simulink model "kalman_estimate_MM"  (R2018b)
settings: Solver=FixedStepAuto  StartTime=0.0  StopTime=500  FixedStep=0.02  RelTol=1e-3
values from neighbouring files (symbols this model uses):
  D = randn(num_output,num_control)    [Com_of_linear_model_calculate.m]    (also in Copy_of_linear_model_calculate.m; D.mat = [0 0 0.00507528406191 0.0236369284061 0.221173094143 0.00198; LINEAR.m = randn(8,1)*10; MM_HKF.m = reshape(out(A_l+B_l+C_l+1:A_l+B_l+C_l+D_l),size_D))
undefined symbols (not defined in the file or in its folder): act_piece, com_piece, piece, sigbuilder_block
libraries: sharedschedule x467, dspsigattribs x44, commchan3 x1
(part 4 of 5)

== system kalman_estimate_MM/sen3_PWL-model ==
  u : Inport
  x0 : Inport  Port=2
  A : sharedschedule/Interpolate Matrix(x)   matrix=sen3_piece.A  aMode=aMode
      settings: SourceProductName=Aerospace Blockset  SourceProductBaseCode=AE
  Add : Sum
  B : sharedschedule/Interpolate Matrix(x)   matrix=sen3_piece.B  aMode=aMode
      settings: SourceProductName=Aerospace Blockset  SourceProductBaseCode=AE
  C : sharedschedule/Interpolate Matrix(x)   matrix=sen3_piece.C  aMode=aMode
      settings: SourceProductName=Aerospace Blockset  SourceProductBaseCode=AE
  D : sharedschedule/Interpolate Matrix(x)   matrix=sen3_piece.D  aMode=aMode
      settings: SourceProductName=Aerospace Blockset  SourceProductBaseCode=AE
  K : sharedschedule/Interpolate Matrix(x)   matrix=sen3_piece.K  aMode=aMode
      settings: SourceProductName=Aerospace Blockset  SourceProductBaseCode=AE
  Minus1 : Sum  Inputs=+-
  Prelookup : PreLookup  BreakpointsData=sen3_piece.Nl  BreakpointObject=Nl  ExtrapMethod=Linear  UseLastBreakpoint=on  DiagnosticForOutOfRangeInput=Warning
  S : sharedschedule/Interpolate Matrix(x)   matrix=sen3_piece.S  aMode=aMode
      settings: SourceProductName=Aerospace Blockset  SourceProductBaseCode=AE
  Selector : Selector  InputPortWidth=2  IndexOptions=Index vector (dialog)  Indices=[1]  OutputSizes=1
  kalman filter1 : Subsystem
  steadyOutput : sharedschedule/Interpolate Matrix(x)   matrix=sen3_piece.steadyOutput  aMode=aMode
      settings: SourceProductName=Aerospace Blockset  SourceProductBaseCode=AE
  steadyState : sharedschedule/Interpolate Matrix(x)   matrix=sen3_piece.steadyState  aMode=aMode
      settings: SourceProductName=Aerospace Blockset  SourceProductBaseCode=AE
  steadyinput : sharedschedule/Interpolate Matrix(x)   matrix=sen3_piece.steadyInput  aMode=aMode
      settings: SourceProductName=Aerospace Blockset  SourceProductBaseCode=AE
  Out1 : Outport
  Out2 : Outport  Port=2
  wires:
  Add/1 -> Out2/1
  steadyOutput/1 -> Add/2
  u/1 -> Minus1/1
  x0/1 -> kalman filter1/5(x0)
  A/1 -> kalman filter1/1(A)
  steadyinput/1 -> Minus1/2
  kalman filter1/1(X_es) -> Selector/1
  Minus1/1 -> kalman filter1/6(U)
  kalman filter1/2(Y_es) -> Out1/1, Add/1
  C/1 -> kalman filter1/3(C)
  steadyState/1 -> kalman filter1/7(Xtrim)
  Selector/1 -> Prelookup/1
  Prelookup/2 -> B/2, C/2, D/2, steadyOutput/2, steadyinput/2, K/2, S/2, steadyState/2, A/2
  B/1 -> kalman filter1/2(B)
  Prelookup/1 -> A/1, B/1, C/1, D/1, steadyOutput/1, steadyinput/1, steadyState/1, K/1, S/1
  D/1 -> kalman filter1/4(D)

== system kalman_estimate_MM/sen8_PIECE kalman ==
  u : Inport
  y : Inport  Port=2
  x0 : Inport  Port=3
  A : sharedschedule/Interpolate Matrix(x)   matrix=sen8_piece.A  aMode=aMode
      settings: SourceProductName=Aerospace Blockset  SourceProductBaseCode=AE
  B : sharedschedule/Interpolate Matrix(x)   matrix=sen8_piece.B  aMode=aMode
      settings: SourceProductName=Aerospace Blockset  SourceProductBaseCode=AE
  C : sharedschedule/Interpolate Matrix(x)   matrix=sen8_piece.C  aMode=aMode
      settings: SourceProductName=Aerospace Blockset  SourceProductBaseCode=AE
  D : sharedschedule/Interpolate Matrix(x)   matrix=sen8_piece.D  aMode=aMode
      settings: SourceProductName=Aerospace Blockset  SourceProductBaseCode=AE
  K_s : sharedschedule/Interpolate Matrix(x)   matrix=sen8_piece.K  aMode=aMode
      settings: SourceProductName=Aerospace Blockset  SourceProductBaseCode=AE
  MATLAB Function : MATLAB Function  TreatAsAtomicUnit=on
  Minus1 : Sum  Inputs=+-
  Minus5 : Sum  Inputs=+-
  Prelookup : PreLookup  BreakpointsData=sen8_piece.Nl  BreakpointObject=Nl  ExtrapMethod=Linear  UseLastBreakpoint=on  DiagnosticForOutOfRangeInput=Warning
  S : sharedschedule/Interpolate Matrix(x)   matrix=sen8_piece.S  aMode=aMode
      settings: SourceProductName=Aerospace Blockset  SourceProductBaseCode=AE
  Selector : Selector  InputPortWidth=2  IndexOptions=Index vector (dialog)  Indices=[1]  OutputSizes=1
  kalman filter1 : Subsystem
  steadyOutput : sharedschedule/Interpolate Matrix(x)   matrix=sen8_piece.steadyOutput  aMode=aMode
      settings: SourceProductName=Aerospace Blockset  SourceProductBaseCode=AE
  steadyState : sharedschedule/Interpolate Matrix(x)   matrix=sen8_piece.steadyState  aMode=aMode
      settings: SourceProductName=Aerospace Blockset  SourceProductBaseCode=AE
  steadyinput : sharedschedule/Interpolate Matrix(x)   matrix=sen8_piece.steadyInput  aMode=aMode
      settings: SourceProductName=Aerospace Blockset  SourceProductBaseCode=AE
  Out1 : Outport
  Out2 : Outport  Port=2
  Out3 : Outport  Port=3
  wires:
  kalman filter1/3(Y_error) -> MATLAB Function/1(err), Out2/1
  u/1 -> Minus1/1
  y/1 -> Minus5/1
  x0/1 -> kalman filter1/6(x0)
  A/1 -> kalman filter1/1(A)
  steadyOutput/1 -> Minus5/2
  K_s/1 -> kalman filter1/5(K)
  steadyinput/1 -> Minus1/2
  kalman filter1/1(X_es) -> Selector/1
  Minus1/1 -> kalman filter1/8(U)
  kalman filter1/2(Y_es) -> Out1/1
  Minus5/1 -> kalman filter1/7(Y)
  C/1 -> kalman filter1/3(C)
  steadyState/1 -> kalman filter1/9(Xtrim)
  Selector/1 -> Prelookup/1
  Prelookup/2 -> B/2, C/2, D/2, steadyOutput/2, steadyinput/2, K_s/2, S/2, steadyState/2, A/2
  B/1 -> kalman filter1/2(B)
  Prelookup/1 -> A/1, B/1, C/1, D/1, steadyOutput/1, steadyinput/1, steadyState/1, K_s/1, S/1
  D/1 -> kalman filter1/4(D)
  S/1 -> MATLAB Function/2(S)
  MATLAB Function/1(y) -> Out3/1

== system kalman_estimate_MM/sen8_PWL ==
  u : Inport
  x0 : Inport  Port=2
  A : sharedschedule/Interpolate Matrix(x)   matrix=sen8_piece.A  aMode=aMode
      settings: SourceProductName=Aerospace Blockset  SourceProductBaseCode=AE
  Add : Sum
  B : sharedschedule/Interpolate Matrix(x)   matrix=sen8_piece.B  aMode=aMode
      settings: SourceProductName=Aerospace Blockset  SourceProductBaseCode=AE
  C : sharedschedule/Interpolate Matrix(x)   matrix=sen8_piece.C  aMode=aMode
      settings: SourceProductName=Aerospace Blockset  SourceProductBaseCode=AE
  D : sharedschedule/Interpolate Matrix(x)   matrix=sen8_piece.D  aMode=aMode
      settings: SourceProductName=Aerospace Blockset  SourceProductBaseCode=AE
  K : sharedschedule/Interpolate Matrix(x)   matrix=sen8_piece.K  aMode=aMode
      settings: SourceProductName=Aerospace Blockset  SourceProductBaseCode=AE
  Minus1 : Sum  Inputs=+-
  Prelookup : PreLookup  BreakpointsData=sen8_piece.Nl  BreakpointObject=Nl  ExtrapMethod=Linear  UseLastBreakpoint=on  DiagnosticForOutOfRangeInput=Warning
  S : sharedschedule/Interpolate Matrix(x)   matrix=sen8_piece.S  aMode=aMode
      settings: SourceProductName=Aerospace Blockset  SourceProductBaseCode=AE
  Selector : Selector  InputPortWidth=2  IndexOptions=Index vector (dialog)  Indices=[1]  OutputSizes=1
  kalman filter1 : Subsystem
  steadyOutput : sharedschedule/Interpolate Matrix(x)   matrix=sen8_piece.steadyOutput  aMode=aMode
      settings: SourceProductName=Aerospace Blockset  SourceProductBaseCode=AE
  steadyState : sharedschedule/Interpolate Matrix(x)   matrix=sen8_piece.steadyState  aMode=aMode
      settings: SourceProductName=Aerospace Blockset  SourceProductBaseCode=AE
  steadyinput : sharedschedule/Interpolate Matrix(x)   matrix=sen8_piece.steadyInput  aMode=aMode
      settings: SourceProductName=Aerospace Blockset  SourceProductBaseCode=AE
  Out1 : Outport
  Out2 : Outport  Port=2
  wires:
  Add/1 -> Out2/1
  steadyOutput/1 -> Add/2
  u/1 -> Minus1/1
  x0/1 -> kalman filter1/5(x0)
  A/1 -> kalman filter1/1(A)
  steadyinput/1 -> Minus1/2
  kalman filter1/1(X_es) -> Selector/1
  Minus1/1 -> kalman filter1/6(U)
  kalman filter1/2(Y_es) -> Out1/1, Add/1
  C/1 -> kalman filter1/3(C)
  steadyState/1 -> kalman filter1/7(Xtrim)
  Selector/1 -> Prelookup/1
  Prelookup/2 -> B/2, D/2, steadyOutput/2, steadyinput/2, K/2, S/2, steadyState/2, C/2, A/2
  B/1 -> kalman filter1/2(B)
  Prelookup/1 -> A/1, B/1, D/1, steadyOutput/1, steadyinput/1, steadyState/1, K/1, S/1, C/1
  D/1 -> kalman filter1/4(D)

== system kalman_estimate_MM/AKF1/kalman  ==
  A : Inport
  C : Inport  Port=2
  K : Inport  Port=3
  x0 : Inport  Port=4
  Y : Inport  Port=5
  Xtrim : Inport  Port=6
  "\tCX" : Product  Multiplication=Matrix(*)
  AX : Product  Multiplication=Matrix(*)
  Delay : Delay  DelayLength=1  InitialConditionSource=Input port
      settings: InputPortMap=u0,p4
  KY : Product  Multiplication=Matrix(*)
  Minus : Sum  Inputs=+-
  Minus1 : Sum
  Minus2 : Sum  Inputs=+-
  Minus3 : Sum
  X_es : Outport
  Y_es : Outport  Port=2
  wires:
  "\tCX"/1 -> Y_es/1, Minus2/2
  KY/1 -> Minus3/1
  Y/1 -> Minus2/1
  x0/1 -> Delay/2
  Minus2/1 -> KY/2
  A/1 -> AX/1
  C/1 -> "\tCX"/1
  K/1 -> KY/1
  Xtrim/1 -> Minus1/2, Minus/2
  Delay/1 -> X_es/1, Minus/1
  Minus/1 -> AX/2, "\tCX"/2
  AX/1 -> Minus3/2
  Minus3/1 -> Minus1/1
  Minus1/1 -> Delay/1

== system kalman_estimate_MM/AKF10/kalman  ==
  A : Inport
  C : Inport  Port=2
  K : Inport  Port=3
  x0 : Inport  Port=4
  Y : Inport  Port=5
  Xtrim : Inport  Port=6
  "\tCX" : Product  Multiplication=Matrix(*)
  AX : Product  Multiplication=Matrix(*)
  Delay : Delay  DelayLength=1  InitialConditionSource=Input port
      settings: InputPortMap=u0,p4
  KY : Product  Multiplication=Matrix(*)
  Minus : Sum  Inputs=+-
  Minus1 : Sum
  Minus2 : Sum  Inputs=+-
  Minus3 : Sum
  X_es : Outport
  Y_es : Outport  Port=2
  wires:
  "\tCX"/1 -> Y_es/1, Minus2/2
  KY/1 -> Minus3/1
  Y/1 -> Minus2/1
  x0/1 -> Delay/2
  Minus2/1 -> KY/2
  A/1 -> AX/1
  C/1 -> "\tCX"/1
  K/1 -> KY/1
  Xtrim/1 -> Minus1/2, Minus/2
  Delay/1 -> X_es/1, Minus/1
  Minus/1 -> AX/2, "\tCX"/2
  AX/1 -> Minus3/2
  Minus3/1 -> Minus1/1
  Minus1/1 -> Delay/1

== system kalman_estimate_MM/AKF12/kalman  ==
  A : Inport
  C : Inport  Port=2
  K : Inport  Port=3
  x0 : Inport  Port=4
  Y : Inport  Port=5
  Xtrim : Inport  Port=6
  "\tCX" : Product  Multiplication=Matrix(*)
  AX : Product  Multiplication=Matrix(*)
  Delay : Delay  DelayLength=1  InitialConditionSource=Input port
      settings: InputPortMap=u0,p4
  KY : Product  Multiplication=Matrix(*)
  Minus : Sum  Inputs=+-
  Minus1 : Sum
  Minus2 : Sum  Inputs=+-
  Minus3 : Sum
  X_es : Outport
  Y_es : Outport  Port=2
  wires:
  Minus1/1 -> Delay/1
  Minus3/1 -> Minus1/1
  AX/1 -> Minus3/2
  Minus/1 -> "\tCX"/2, AX/2
  Delay/1 -> Minus/1, X_es/1
  Xtrim/1 -> Minus/2, Minus1/2
  K/1 -> KY/1
  C/1 -> "\tCX"/1
  A/1 -> AX/1
  Minus2/1 -> KY/2
  x0/1 -> Delay/2
  Y/1 -> Minus2/1
  KY/1 -> Minus3/1
  "\tCX"/1 -> Minus2/2, Y_es/1

== system kalman_estimate_MM/AKF2/kalman  ==
  A : Inport
  C : Inport  Port=2
  K : Inport  Port=3
  x0 : Inport  Port=4
  Y : Inport  Port=5
  Xtrim : Inport  Port=6
  "\tCX" : Product  Multiplication=Matrix(*)
  AX : Product  Multiplication=Matrix(*)
  Delay : Delay  DelayLength=1  InitialConditionSource=Input port
      settings: InputPortMap=u0,p4
  KY : Product  Multiplication=Matrix(*)
  Minus : Sum  Inputs=+-
  Minus1 : Sum
  Minus2 : Sum  Inputs=+-
  Minus3 : Sum
  X_es : Outport
  Y_es : Outport  Port=2
  wires:
  Minus1/1 -> Delay/1
  Minus3/1 -> Minus1/1
  AX/1 -> Minus3/2
  Minus/1 -> "\tCX"/2, AX/2
  Delay/1 -> Minus/1, X_es/1
  Xtrim/1 -> Minus/2, Minus1/2
  K/1 -> KY/1
  C/1 -> "\tCX"/1
  A/1 -> AX/1
  Minus2/1 -> KY/2
  x0/1 -> Delay/2
  Y/1 -> Minus2/1
  KY/1 -> Minus3/1
  "\tCX"/1 -> Minus2/2, Y_es/1

== system kalman_estimate_MM/AKF3/kalman  ==
  A : Inport
  C : Inport  Port=2
  K : Inport  Port=3
  x0 : Inport  Port=4
  Y : Inport  Port=5
  Xtrim : Inport  Port=6
  "\tCX" : Product  Multiplication=Matrix(*)
  AX : Product  Multiplication=Matrix(*)
  Delay : Delay  DelayLength=1  InitialConditionSource=Input port
      settings: InputPortMap=u0,p4
  KY : Product  Multiplication=Matrix(*)
  Minus : Sum  Inputs=+-
  Minus1 : Sum
  Minus2 : Sum  Inputs=+-
  Minus3 : Sum
  X_es : Outport
  Y_es : Outport  Port=2
  wires:
  "\tCX"/1 -> Y_es/1, Minus2/2
  KY/1 -> Minus3/1
  Y/1 -> Minus2/1
  x0/1 -> Delay/2
  Minus2/1 -> KY/2
  A/1 -> AX/1
  C/1 -> "\tCX"/1
  K/1 -> KY/1
  Xtrim/1 -> Minus1/2, Minus/2
  Delay/1 -> X_es/1, Minus/1
  Minus/1 -> AX/2, "\tCX"/2
  AX/1 -> Minus3/2
  Minus3/1 -> Minus1/1
  Minus1/1 -> Delay/1

== system kalman_estimate_MM/AKF4/kalman  ==
  A : Inport
  C : Inport  Port=2
  K : Inport  Port=3
  x0 : Inport  Port=4
  Y : Inport  Port=5
  Xtrim : Inport  Port=6
  "\tCX" : Product  Multiplication=Matrix(*)
  AX : Product  Multiplication=Matrix(*)
  Delay : Delay  DelayLength=1  InitialConditionSource=Input port
      settings: InputPortMap=u0,p4
  KY : Product  Multiplication=Matrix(*)
  Minus : Sum  Inputs=+-
  Minus1 : Sum
  Minus2 : Sum  Inputs=+-
  Minus3 : Sum
  X_es : Outport
  Y_es : Outport  Port=2
  wires:
  Minus1/1 -> Delay/1
  Minus3/1 -> Minus1/1
  AX/1 -> Minus3/2
  Minus/1 -> "\tCX"/2, AX/2
  Delay/1 -> Minus/1, X_es/1
  Xtrim/1 -> Minus/2, Minus1/2
  K/1 -> KY/1
  C/1 -> "\tCX"/1
  A/1 -> AX/1
  Minus2/1 -> KY/2
  x0/1 -> Delay/2
  Y/1 -> Minus2/1
  KY/1 -> Minus3/1
  "\tCX"/1 -> Minus2/2, Y_es/1

== system kalman_estimate_MM/AKF5/kalman  ==
  A : Inport
  C : Inport  Port=2
  K : Inport  Port=3
  x0 : Inport  Port=4
  Y : Inport  Port=5
  Xtrim : Inport  Port=6
  "\tCX" : Product  Multiplication=Matrix(*)
  AX : Product  Multiplication=Matrix(*)
  Delay : Delay  DelayLength=1  InitialConditionSource=Input port
      settings: InputPortMap=u0,p4
  KY : Product  Multiplication=Matrix(*)
  Minus : Sum  Inputs=+-
  Minus1 : Sum
  Minus2 : Sum  Inputs=+-
  Minus3 : Sum
  X_es : Outport
  Y_es : Outport  Port=2
  wires:
  "\tCX"/1 -> Y_es/1, Minus2/2
  KY/1 -> Minus3/1
  Y/1 -> Minus2/1
  x0/1 -> Delay/2
  Minus2/1 -> KY/2
  A/1 -> AX/1
  C/1 -> "\tCX"/1
  K/1 -> KY/1
  Xtrim/1 -> Minus1/2, Minus/2
  Delay/1 -> X_es/1, Minus/1
  Minus/1 -> AX/2, "\tCX"/2
  AX/1 -> Minus3/2
  Minus3/1 -> Minus1/1
  Minus1/1 -> Delay/1

== system kalman_estimate_MM/AKF6/kalman  ==
  A : Inport
  C : Inport  Port=2
  K : Inport  Port=3
  x0 : Inport  Port=4
  Y : Inport  Port=5
  Xtrim : Inport  Port=6
  "\tCX" : Product  Multiplication=Matrix(*)
  AX : Product  Multiplication=Matrix(*)
  Delay : Delay  DelayLength=1  InitialConditionSource=Input port
      settings: InputPortMap=u0,p4
  KY : Product  Multiplication=Matrix(*)
  Minus : Sum  Inputs=+-
  Minus1 : Sum
  Minus2 : Sum  Inputs=+-
  Minus3 : Sum
  X_es : Outport
  Y_es : Outport  Port=2
  wires:
  Minus1/1 -> Delay/1
  Minus3/1 -> Minus1/1
  AX/1 -> Minus3/2
  Minus/1 -> "\tCX"/2, AX/2
  Delay/1 -> Minus/1, X_es/1
  Xtrim/1 -> Minus/2, Minus1/2
  K/1 -> KY/1
  C/1 -> "\tCX"/1
  A/1 -> AX/1
  Minus2/1 -> KY/2
  x0/1 -> Delay/2
  Y/1 -> Minus2/1
  KY/1 -> Minus3/1
  "\tCX"/1 -> Minus2/2, Y_es/1

== system kalman_estimate_MM/AKF7/kalman  ==
  A : Inport
  C : Inport  Port=2
  K : Inport  Port=3
  x0 : Inport  Port=4
  Y : Inport  Port=5
  Xtrim : Inport  Port=6
  "\tCX" : Product  Multiplication=Matrix(*)
  AX : Product  Multiplication=Matrix(*)
  Delay : Delay  DelayLength=1  InitialConditionSource=Input port
      settings: InputPortMap=u0,p4
  KY : Product  Multiplication=Matrix(*)
  Minus : Sum  Inputs=+-
  Minus1 : Sum
  Minus2 : Sum  Inputs=+-
  Minus3 : Sum
  X_es : Outport
  Y_es : Outport  Port=2
  wires:
  "\tCX"/1 -> Y_es/1, Minus2/2
  KY/1 -> Minus3/1
  Y/1 -> Minus2/1
  x0/1 -> Delay/2
  Minus2/1 -> KY/2
  A/1 -> AX/1
  C/1 -> "\tCX"/1
  K/1 -> KY/1
  Xtrim/1 -> Minus1/2, Minus/2
  Delay/1 -> X_es/1, Minus/1
  Minus/1 -> AX/2, "\tCX"/2
  AX/1 -> Minus3/2
  Minus3/1 -> Minus1/1
  Minus1/1 -> Delay/1

== system kalman_estimate_MM/AKF8/kalman  ==
  A : Inport
  C : Inport  Port=2
  K : Inport  Port=3
  x0 : Inport  Port=4
  Y : Inport  Port=5
  Xtrim : Inport  Port=6
  "\tCX" : Product  Multiplication=Matrix(*)
  AX : Product  Multiplication=Matrix(*)
  Delay : Delay  DelayLength=1  InitialConditionSource=Input port
      settings: InputPortMap=u0,p4
  KY : Product  Multiplication=Matrix(*)
  Minus : Sum  Inputs=+-
  Minus1 : Sum
  Minus2 : Sum  Inputs=+-
  Minus3 : Sum
  X_es : Outport
  Y_es : Outport  Port=2
  wires:
  Minus1/1 -> Delay/1
  Minus3/1 -> Minus1/1
  AX/1 -> Minus3/2
  Minus/1 -> "\tCX"/2, AX/2
  Delay/1 -> Minus/1, X_es/1
  Xtrim/1 -> Minus/2, Minus1/2
  K/1 -> KY/1
  C/1 -> "\tCX"/1
  A/1 -> AX/1
  Minus2/1 -> KY/2
  x0/1 -> Delay/2
  Y/1 -> Minus2/1
  KY/1 -> Minus3/1
  "\tCX"/1 -> Minus2/2, Y_es/1

== system kalman_estimate_MM/AKF9/kalman  ==
  A : Inport
  C : Inport  Port=2
  K : Inport  Port=3
  x0 : Inport  Port=4
  Y : Inport  Port=5
  Xtrim : Inport  Port=6
  "\tCX" : Product  Multiplication=Matrix(*)
  AX : Product  Multiplication=Matrix(*)
  Delay : Delay  DelayLength=1  InitialConditionSource=Input port
      settings: InputPortMap=u0,p4
  KY : Product  Multiplication=Matrix(*)
  Minus : Sum  Inputs=+-
  Minus1 : Sum
  Minus2 : Sum  Inputs=+-
  Minus3 : Sum
  X_es : Outport
  Y_es : Outport  Port=2
  wires:
  "\tCX"/1 -> Y_es/1, Minus2/2
  KY/1 -> Minus3/1
  Y/1 -> Minus2/1
  x0/1 -> Delay/2
  Minus2/1 -> KY/2
  A/1 -> AX/1
  C/1 -> "\tCX"/1
  K/1 -> KY/1
  Xtrim/1 -> Minus1/2, Minus/2
  Delay/1 -> X_es/1, Minus/1
  Minus/1 -> AX/2, "\tCX"/2
  AX/1 -> Minus3/2
  Minus3/1 -> Minus1/1
  Minus1/1 -> Delay/1

== system kalman_estimate_MM/HKF1/kalman filter1 ==
  A : Inport
  C : Inport  Port=2
  K : Inport  Port=3
  x0 : Inport  Port=4
  Y : Inport  Port=5
  Xtrim : Inport  Port=6
  L : Inport  Port=7
  M : Inport  Port=8
  P : Inport  Port=9
  "\tCX" : Product  Multiplication=Matrix(*)
  AX : Product  Multiplication=Matrix(*)
  Convert 1-D to 2-D : dspsigattribs/Convert 1-D to 2-D  M=10  N=1  frameBasedOut=off
      settings: SourceProductName=DSP System Toolbox  SourceProductBaseCode=DS
  Convert 1-D to 2-D1 : dspsigattribs/Convert 1-D to 2-D  M=2  N=1  frameBasedOut=off
      settings: SourceProductName=DSP System Toolbox  SourceProductBaseCode=DS
  Delay : Delay  DelayLength=1  InitialConditionSource=Input port
      settings: InputPortMap=u0,p4
  KY : Product  Multiplication=Matrix(*)
  LP : Product  Multiplication=Matrix(*)
  MATLAB Function : MATLAB Function  TreatAsAtomicUnit=on
  MP : Product  Multiplication=Matrix(*)
  Minus : Sum  Inputs=+-
  Minus1 : Sum
  Minus2 : Sum  Inputs=+-
  Minus3 : Sum  Inputs=+++
  Minus4 : Sum
  X_es : Outport
  Y_es : Outport  Port=2
  Y_error : Outport  Port=3
  wires:
  MATLAB Function/1(y) -> KY/2, Y_error/1
  Minus2/1 -> MATLAB Function/1(u)
  Convert 1-D to 2-D1/1 -> Delay/2
  x0/1 -> Convert 1-D to 2-D1/1
  Convert 1-D to 2-D/1 -> MP/2, LP/2
  P/1 -> Convert 1-D to 2-D/1
  MP/1 -> Minus4/2
  LP/1 -> Minus3/3
  M/1 -> MP/1
  L/1 -> LP/1
  Minus4/1 -> Minus2/2, Y_es/1
  KY/1 -> Minus3/1
  Y/1 -> Minus2/1
  "\tCX"/1 -> Minus4/1
  A/1 -> AX/1
  C/1 -> "\tCX"/1
  K/1 -> KY/1
  Xtrim/1 -> Minus1/2, Minus/2
  Delay/1 -> Minus/1, X_es/1
  Minus/1 -> AX/2, "\tCX"/2
  AX/1 -> Minus3/2
  Minus3/1 -> Minus1/1
  Minus1/1 -> Delay/1

== system kalman_estimate_MM/HKF10/kalman filter1 ==
  A : Inport
  C : Inport  Port=2
  x0 : Inport  Port=3
  Xtrim : Inport  Port=4
  L : Inport  Port=5
  M : Inport  Port=6
  P : Inport  Port=7
  "\tCX" : Product  Multiplication=Matrix(*)
  AX : Product  Multiplication=Matrix(*)
  Convert 1-D to 2-D : dspsigattribs/Convert 1-D to 2-D  M=10  N=1  frameBasedOut=off
      settings: SourceProductName=DSP System Toolbox  SourceProductBaseCode=DS
  Convert 1-D to 2-D1 : dspsigattribs/Convert 1-D to 2-D  M=2  N=1  frameBasedOut=off
      settings: SourceProductName=DSP System Toolbox  SourceProductBaseCode=DS
  Delay : Delay  DelayLength=1  InitialConditionSource=Input port
      settings: InputPortMap=u0,p4
  LP : Product  Multiplication=Matrix(*)
  MP : Product  Multiplication=Matrix(*)
  Minus : Sum  Inputs=+-
  Minus1 : Sum
  Minus3 : Sum
  Minus4 : Sum
  X_es : Outport
  Y_es : Outport  Port=2
  wires:
  Minus1/1 -> Delay/1
  Minus3/1 -> Minus1/1
  AX/1 -> Minus3/2
  Minus/1 -> "\tCX"/2, AX/2
  Delay/1 -> X_es/1, Minus/1
  Xtrim/1 -> Minus/2, Minus1/2
  C/1 -> "\tCX"/1
  A/1 -> AX/1
  "\tCX"/1 -> Minus4/1
  Minus4/1 -> Y_es/1
  L/1 -> LP/1
  M/1 -> MP/1
  LP/1 -> Minus3/1
  MP/1 -> Minus4/2
  P/1 -> Convert 1-D to 2-D/1
  Convert 1-D to 2-D/1 -> LP/2, MP/2
  x0/1 -> Convert 1-D to 2-D1/1
  Convert 1-D to 2-D1/1 -> Delay/2

== system kalman_estimate_MM/HKF11/kalman filter1 ==
  A : Inport
  C : Inport  Port=2
  x0 : Inport  Port=3
  Xtrim : Inport  Port=4
  L : Inport  Port=5
  M : Inport  Port=6
  P : Inport  Port=7
  "\tCX" : Product  Multiplication=Matrix(*)
  AX : Product  Multiplication=Matrix(*)
  Convert 1-D to 2-D : dspsigattribs/Convert 1-D to 2-D  M=10  N=1  frameBasedOut=off
      settings: SourceProductName=DSP System Toolbox  SourceProductBaseCode=DS
  Convert 1-D to 2-D1 : dspsigattribs/Convert 1-D to 2-D  M=2  N=1  frameBasedOut=off
      settings: SourceProductName=DSP System Toolbox  SourceProductBaseCode=DS
  Delay : Delay  DelayLength=1  InitialConditionSource=Input port
      settings: InputPortMap=u0,p4
  LP : Product  Multiplication=Matrix(*)
  MP : Product  Multiplication=Matrix(*)
  Minus : Sum  Inputs=+-
  Minus1 : Sum
  Minus3 : Sum
  Minus4 : Sum
  X_es : Outport
  Y_es : Outport  Port=2
  wires:
  Convert 1-D to 2-D1/1 -> Delay/2
  x0/1 -> Convert 1-D to 2-D1/1
  Convert 1-D to 2-D/1 -> MP/2, LP/2
  P/1 -> Convert 1-D to 2-D/1
  MP/1 -> Minus4/2
  LP/1 -> Minus3/1
  M/1 -> MP/1
  L/1 -> LP/1
  Minus4/1 -> Y_es/1
  "\tCX"/1 -> Minus4/1
  A/1 -> AX/1
  C/1 -> "\tCX"/1
  Xtrim/1 -> Minus1/2, Minus/2
  Delay/1 -> Minus/1, X_es/1
  Minus/1 -> AX/2, "\tCX"/2
  AX/1 -> Minus3/2
  Minus3/1 -> Minus1/1
  Minus1/1 -> Delay/1

== system kalman_estimate_MM/HKF2/kalman filter1 ==
  A : Inport
  C : Inport  Port=2
  x0 : Inport  Port=3
  Xtrim : Inport  Port=4
  L : Inport  Port=5
  M : Inport  Port=6
  P : Inport  Port=7
  "\tCX" : Product  Multiplication=Matrix(*)
  AX : Product  Multiplication=Matrix(*)
  Convert 1-D to 2-D : dspsigattribs/Convert 1-D to 2-D  M=10  N=1  frameBasedOut=off
      settings: SourceProductName=DSP System Toolbox  SourceProductBaseCode=DS
  Convert 1-D to 2-D1 : dspsigattribs/Convert 1-D to 2-D  M=2  N=1  frameBasedOut=off
      settings: SourceProductName=DSP System Toolbox  SourceProductBaseCode=DS
  Delay : Delay  DelayLength=1  InitialConditionSource=Input port
      settings: InputPortMap=u0,p4
  LP : Product  Multiplication=Matrix(*)
  MP : Product  Multiplication=Matrix(*)
  Minus : Sum  Inputs=+-
  Minus1 : Sum
  Minus3 : Sum
  Minus4 : Sum
  X_es : Outport
  Y_es : Outport  Port=2
  wires:
  Convert 1-D to 2-D1/1 -> Delay/2
  x0/1 -> Convert 1-D to 2-D1/1
  Convert 1-D to 2-D/1 -> MP/2, LP/2
  P/1 -> Convert 1-D to 2-D/1
  MP/1 -> Minus4/2
  LP/1 -> Minus3/1
  M/1 -> MP/1
  L/1 -> LP/1
  Minus4/1 -> Y_es/1
  "\tCX"/1 -> Minus4/1
  A/1 -> AX/1
  C/1 -> "\tCX"/1
  Xtrim/1 -> Minus1/2, Minus/2
  Delay/1 -> Minus/1, X_es/1
  Minus/1 -> AX/2, "\tCX"/2
  AX/1 -> Minus3/2
  Minus3/1 -> Minus1/1
  Minus1/1 -> Delay/1

== system kalman_estimate_MM/HKF3/kalman filter1 ==
  A : Inport
  C : Inport  Port=2
  K : Inport  Port=3
  x0 : Inport  Port=4
  Y : Inport  Port=5
  Xtrim : Inport  Port=6
  L : Inport  Port=7
  M : Inport  Port=8
  P : Inport  Port=9
  "\tCX" : Product  Multiplication=Matrix(*)
  AX : Product  Multiplication=Matrix(*)
  Convert 1-D to 2-D : dspsigattribs/Convert 1-D to 2-D  M=10  N=1  frameBasedOut=off
      settings: SourceProductName=DSP System Toolbox  SourceProductBaseCode=DS
  Convert 1-D to 2-D1 : dspsigattribs/Convert 1-D to 2-D  M=2  N=1  frameBasedOut=off
      settings: SourceProductName=DSP System Toolbox  SourceProductBaseCode=DS
  Delay : Delay  DelayLength=1  InitialConditionSource=Input port
      settings: InputPortMap=u0,p4
  KY : Product  Multiplication=Matrix(*)
  LP : Product  Multiplication=Matrix(*)
  MATLAB Function : MATLAB Function  TreatAsAtomicUnit=on
  MP : Product  Multiplication=Matrix(*)
  Minus : Sum  Inputs=+-
  Minus1 : Sum
  Minus2 : Sum  Inputs=+-
  Minus3 : Sum  Inputs=+++
  Minus4 : Sum
  X_es : Outport
  Y_es : Outport  Port=2
  Y_error : Outport  Port=3
  wires:
  MATLAB Function/1(y) -> KY/2, Y_error/1
  Minus2/1 -> MATLAB Function/1(u)
  Convert 1-D to 2-D1/1 -> Delay/2
  x0/1 -> Convert 1-D to 2-D1/1
  Convert 1-D to 2-D/1 -> MP/2, LP/2
  P/1 -> Convert 1-D to 2-D/1
  MP/1 -> Minus4/2
  LP/1 -> Minus3/3
  M/1 -> MP/1
  L/1 -> LP/1
  Minus4/1 -> Minus2/2, Y_es/1
  KY/1 -> Minus3/1
  Y/1 -> Minus2/1
  "\tCX"/1 -> Minus4/1
  A/1 -> AX/1
  C/1 -> "\tCX"/1
  K/1 -> KY/1
  Xtrim/1 -> Minus1/2, Minus/2
  Delay/1 -> Minus/1, X_es/1
  Minus/1 -> AX/2, "\tCX"/2
  AX/1 -> Minus3/2
  Minus3/1 -> Minus1/1
  Minus1/1 -> Delay/1

== system kalman_estimate_MM/HKF4/kalman filter1 ==
  A : Inport
  C : Inport  Port=2
  K : Inport  Port=3
  x0 : Inport  Port=4
  Y : Inport  Port=5
  Xtrim : Inport  Port=6
  L : Inport  Port=7
  M : Inport  Port=8
  P : Inport  Port=9
  "\tCX" : Product  Multiplication=Matrix(*)
  AX : Product  Multiplication=Matrix(*)
  Convert 1-D to 2-D : dspsigattribs/Convert 1-D to 2-D  M=10  N=1  frameBasedOut=off
      settings: SourceProductName=DSP System Toolbox  SourceProductBaseCode=DS
  Convert 1-D to 2-D1 : dspsigattribs/Convert 1-D to 2-D  M=2  N=1  frameBasedOut=off
      settings: SourceProductName=DSP System Toolbox  SourceProductBaseCode=DS
  Delay : Delay  DelayLength=1  InitialConditionSource=Input port
      settings: InputPortMap=u0,p4
  KY : Product  Multiplication=Matrix(*)
  LP : Product  Multiplication=Matrix(*)
  MATLAB Function : MATLAB Function  TreatAsAtomicUnit=on
  MP : Product  Multiplication=Matrix(*)
  Minus : Sum  Inputs=+-
  Minus1 : Sum
  Minus2 : Sum  Inputs=+-
  Minus3 : Sum  Inputs=+++
  Minus4 : Sum
  X_es : Outport
  Y_es : Outport  Port=2
  Y_error : Outport  Port=3
  wires:
  Minus1/1 -> Delay/1
  Minus3/1 -> Minus1/1
  AX/1 -> Minus3/2
  Minus/1 -> "\tCX"/2, AX/2
  Delay/1 -> X_es/1, Minus/1
  Xtrim/1 -> Minus/2, Minus1/2
  K/1 -> KY/1
  C/1 -> "\tCX"/1
  A/1 -> AX/1
  "\tCX"/1 -> Minus4/1
  Y/1 -> Minus2/1
  KY/1 -> Minus3/1
  Minus4/1 -> Y_es/1, Minus2/2
  L/1 -> LP/1
  M/1 -> MP/1
  LP/1 -> Minus3/3
  MP/1 -> Minus4/2
  P/1 -> Convert 1-D to 2-D/1
  Convert 1-D to 2-D/1 -> LP/2, MP/2
  x0/1 -> Convert 1-D to 2-D1/1
  Convert 1-D to 2-D1/1 -> Delay/2
  Minus2/1 -> MATLAB Function/1(u)
  MATLAB Function/1(y) -> Y_error/1, KY/2

== system kalman_estimate_MM/HKF5/kalman filter1 ==
  A : Inport
  C : Inport  Port=2
  K : Inport  Port=3
  x0 : Inport  Port=4
  Y : Inport  Port=5
  Xtrim : Inport  Port=6
  L : Inport  Port=7
  M : Inport  Port=8
  P : Inport  Port=9
  "\tCX" : Product  Multiplication=Matrix(*)
  AX : Product  Multiplication=Matrix(*)
  Convert 1-D to 2-D : dspsigattribs/Convert 1-D to 2-D  M=10  N=1  frameBasedOut=off
      settings: SourceProductName=DSP System Toolbox  SourceProductBaseCode=DS
  Convert 1-D to 2-D1 : dspsigattribs/Convert 1-D to 2-D  M=2  N=1  frameBasedOut=off
      settings: SourceProductName=DSP System Toolbox  SourceProductBaseCode=DS
  Delay : Delay  DelayLength=1  InitialConditionSource=Input port
      settings: InputPortMap=u0,p4
  KY : Product  Multiplication=Matrix(*)
  LP : Product  Multiplication=Matrix(*)
  MATLAB Function : MATLAB Function  TreatAsAtomicUnit=on
  MP : Product  Multiplication=Matrix(*)
  Minus : Sum  Inputs=+-
  Minus1 : Sum
  Minus2 : Sum  Inputs=+-
  Minus3 : Sum  Inputs=+++
  Minus4 : Sum
  X_es : Outport
  Y_es : Outport  Port=2
  Y_error : Outport  Port=3
  wires:
  MATLAB Function/1(y) -> KY/2, Y_error/1
  Minus2/1 -> MATLAB Function/1(u)
  Convert 1-D to 2-D1/1 -> Delay/2
  x0/1 -> Convert 1-D to 2-D1/1
  Convert 1-D to 2-D/1 -> MP/2, LP/2
  P/1 -> Convert 1-D to 2-D/1
  MP/1 -> Minus4/2
  LP/1 -> Minus3/3
  M/1 -> MP/1
  L/1 -> LP/1
  Minus4/1 -> Minus2/2, Y_es/1
  KY/1 -> Minus3/1
  Y/1 -> Minus2/1
  "\tCX"/1 -> Minus4/1
  A/1 -> AX/1
  C/1 -> "\tCX"/1
  K/1 -> KY/1
  Xtrim/1 -> Minus1/2, Minus/2
  Delay/1 -> Minus/1, X_es/1
  Minus/1 -> AX/2, "\tCX"/2
  AX/1 -> Minus3/2
  Minus3/1 -> Minus1/1
  Minus1/1 -> Delay/1

== system kalman_estimate_MM/HKF6/kalman filter1 ==
  A : Inport
  C : Inport  Port=2
  K : Inport  Port=3
  x0 : Inport  Port=4
  Y : Inport  Port=5
  Xtrim : Inport  Port=6
  L : Inport  Port=7
  M : Inport  Port=8
  P : Inport  Port=9
  "\tCX" : Product  Multiplication=Matrix(*)
  AX : Product  Multiplication=Matrix(*)
  Convert 1-D to 2-D : dspsigattribs/Convert 1-D to 2-D  M=10  N=1  frameBasedOut=off
      settings: SourceProductName=DSP System Toolbox  SourceProductBaseCode=DS
  Convert 1-D to 2-D1 : dspsigattribs/Convert 1-D to 2-D  M=2  N=1  frameBasedOut=off
      settings: SourceProductName=DSP System Toolbox  SourceProductBaseCode=DS
  Delay : Delay  DelayLength=1  InitialConditionSource=Input port
      settings: InputPortMap=u0,p4
  KY : Product  Multiplication=Matrix(*)
  LP : Product  Multiplication=Matrix(*)
  MATLAB Function : MATLAB Function  TreatAsAtomicUnit=on
  MP : Product  Multiplication=Matrix(*)
  Minus : Sum  Inputs=+-
  Minus1 : Sum
  Minus2 : Sum  Inputs=+-
  Minus3 : Sum  Inputs=+++
  Minus4 : Sum
  X_es : Outport
  Y_es : Outport  Port=2
  Y_error : Outport  Port=3
  wires:
  Minus1/1 -> Delay/1
  Minus3/1 -> Minus1/1
  AX/1 -> Minus3/2
  Minus/1 -> "\tCX"/2, AX/2
  Delay/1 -> X_es/1, Minus/1
  Xtrim/1 -> Minus/2, Minus1/2
  K/1 -> KY/1
  C/1 -> "\tCX"/1
  A/1 -> AX/1
  "\tCX"/1 -> Minus4/1
  Y/1 -> Minus2/1
  KY/1 -> Minus3/1
  Minus4/1 -> Y_es/1, Minus2/2
  L/1 -> LP/1
  M/1 -> MP/1
  LP/1 -> Minus3/3
  MP/1 -> Minus4/2
  P/1 -> Convert 1-D to 2-D/1
  Convert 1-D to 2-D/1 -> LP/2, MP/2
  x0/1 -> Convert 1-D to 2-D1/1
  Convert 1-D to 2-D1/1 -> Delay/2
  Minus2/1 -> MATLAB Function/1(u)
  MATLAB Function/1(y) -> Y_error/1, KY/2

== system kalman_estimate_MM/HKF7/kalman filter1 ==
  A : Inport
  C : Inport  Port=2
  K : Inport  Port=3
  x0 : Inport  Port=4
  Y : Inport  Port=5
  Xtrim : Inport  Port=6
  L : Inport  Port=7
  M : Inport  Port=8
  P : Inport  Port=9
  "\tCX" : Product  Multiplication=Matrix(*)
  AX : Product  Multiplication=Matrix(*)
  Convert 1-D to 2-D : dspsigattribs/Convert 1-D to 2-D  M=10  N=1  frameBasedOut=off
      settings: SourceProductName=DSP System Toolbox  SourceProductBaseCode=DS
  Convert 1-D to 2-D1 : dspsigattribs/Convert 1-D to 2-D  M=2  N=1  frameBasedOut=off
      settings: SourceProductName=DSP System Toolbox  SourceProductBaseCode=DS
  Delay : Delay  DelayLength=1  InitialConditionSource=Input port
      settings: InputPortMap=u0,p4
  KY : Product  Multiplication=Matrix(*)
  LP : Product  Multiplication=Matrix(*)
  MATLAB Function : MATLAB Function  TreatAsAtomicUnit=on
  MP : Product  Multiplication=Matrix(*)
  Minus : Sum  Inputs=+-
  Minus1 : Sum
  Minus2 : Sum  Inputs=+-
  Minus3 : Sum  Inputs=+++
  Minus4 : Sum
  X_es : Outport
  Y_es : Outport  Port=2
  Y_error : Outport  Port=3
  wires:
  MATLAB Function/1(y) -> KY/2, Y_error/1
  Minus2/1 -> MATLAB Function/1(u)
  Convert 1-D to 2-D1/1 -> Delay/2
  x0/1 -> Convert 1-D to 2-D1/1
  Convert 1-D to 2-D/1 -> MP/2, LP/2
  P/1 -> Convert 1-D to 2-D/1
  MP/1 -> Minus4/2
  LP/1 -> Minus3/3
  M/1 -> MP/1
  L/1 -> LP/1
  Minus4/1 -> Minus2/2, Y_es/1
  KY/1 -> Minus3/1
  Y/1 -> Minus2/1
  "\tCX"/1 -> Minus4/1
  A/1 -> AX/1
  C/1 -> "\tCX"/1
  K/1 -> KY/1
  Xtrim/1 -> Minus1/2, Minus/2
  Delay/1 -> Minus/1, X_es/1
  Minus/1 -> AX/2, "\tCX"/2
  AX/1 -> Minus3/2
  Minus3/1 -> Minus1/1
  Minus1/1 -> Delay/1

== system kalman_estimate_MM/HKF8/kalman filter1 ==
  A : Inport
  C : Inport  Port=2
  x0 : Inport  Port=3
  Xtrim : Inport  Port=4
  L : Inport  Port=5
  M : Inport  Port=6
  P : Inport  Port=7
  "\tCX" : Product  Multiplication=Matrix(*)
  AX : Product  Multiplication=Matrix(*)
  Convert 1-D to 2-D : dspsigattribs/Convert 1-D to 2-D  M=10  N=1  frameBasedOut=off
      settings: SourceProductName=DSP System Toolbox  SourceProductBaseCode=DS
  Convert 1-D to 2-D1 : dspsigattribs/Convert 1-D to 2-D  M=2  N=1  frameBasedOut=off
      settings: SourceProductName=DSP System Toolbox  SourceProductBaseCode=DS
  Delay : Delay  DelayLength=1  InitialConditionSource=Input port
      settings: InputPortMap=u0,p4
  LP : Product  Multiplication=Matrix(*)
  MP : Product  Multiplication=Matrix(*)
  Minus : Sum  Inputs=+-
  Minus1 : Sum
  Minus3 : Sum
  Minus4 : Sum
  X_es : Outport
  Y_es : Outport  Port=2
  wires:
  Minus1/1 -> Delay/1
  Minus3/1 -> Minus1/1
  AX/1 -> Minus3/2
  Minus/1 -> "\tCX"/2, AX/2
  Delay/1 -> X_es/1, Minus/1
  Xtrim/1 -> Minus/2, Minus1/2
  C/1 -> "\tCX"/1
  A/1 -> AX/1
  "\tCX"/1 -> Minus4/1
  Minus4/1 -> Y_es/1
  L/1 -> LP/1
  M/1 -> MP/1
  LP/1 -> Minus3/1
  MP/1 -> Minus4/2
  P/1 -> Convert 1-D to 2-D/1
  Convert 1-D to 2-D/1 -> LP/2, MP/2
  x0/1 -> Convert 1-D to 2-D1/1
  Convert 1-D to 2-D1/1 -> Delay/2

== system kalman_estimate_MM/HKF9/kalman filter1 ==
  A : Inport
  C : Inport  Port=2
  K : Inport  Port=3
  x0 : Inport  Port=4
  Y : Inport  Port=5
  Xtrim : Inport  Port=6
  L : Inport  Port=7
  M : Inport  Port=8
  P : Inport  Port=9
  "\tCX" : Product  Multiplication=Matrix(*)
  AX : Product  Multiplication=Matrix(*)
  Convert 1-D to 2-D : dspsigattribs/Convert 1-D to 2-D  M=10  N=1  frameBasedOut=off
      settings: SourceProductName=DSP System Toolbox  SourceProductBaseCode=DS
  Convert 1-D to 2-D1 : dspsigattribs/Convert 1-D to 2-D  M=2  N=1  frameBasedOut=off
      settings: SourceProductName=DSP System Toolbox  SourceProductBaseCode=DS
  Delay : Delay  DelayLength=1  InitialConditionSource=Input port
      settings: InputPortMap=u0,p4
  KY : Product  Multiplication=Matrix(*)
  LP : Product  Multiplication=Matrix(*)
  MATLAB Function : MATLAB Function  TreatAsAtomicUnit=on
  MP : Product  Multiplication=Matrix(*)
  Minus : Sum  Inputs=+-
  Minus1 : Sum
  Minus2 : Sum  Inputs=+-
  Minus3 : Sum  Inputs=+++
  Minus4 : Sum
  X_es : Outport
  Y_es : Outport  Port=2
  Y_error : Outport  Port=3
  wires:
  Minus1/1 -> Delay/1
  Minus3/1 -> Minus1/1
  AX/1 -> Minus3/2
  Minus/1 -> "\tCX"/2, AX/2
  Delay/1 -> X_es/1, Minus/1
  Xtrim/1 -> Minus/2, Minus1/2
  K/1 -> KY/1
  C/1 -> "\tCX"/1
  A/1 -> AX/1
  "\tCX"/1 -> Minus4/1
  Y/1 -> Minus2/1
  KY/1 -> Minus3/1
  Minus4/1 -> Y_es/1, Minus2/2
  L/1 -> LP/1
  M/1 -> MP/1
  LP/1 -> Minus3/3
  MP/1 -> Minus4/2
  P/1 -> Convert 1-D to 2-D/1
  Convert 1-D to 2-D/1 -> LP/2, MP/2
  x0/1 -> Convert 1-D to 2-D1/1
  Convert 1-D to 2-D1/1 -> Delay/2
  Minus2/1 -> MATLAB Function/1(u)
  MATLAB Function/1(y) -> Y_error/1, KY/2

== system kalman_estimate_MM/PIECE kalman/kalman filter1 ==
  A : Inport
  B : Inport  Port=2
  C : Inport  Port=3
  D : Inport  Port=4
  K : Inport  Port=5
  x0 : Inport  Port=6
  Y : Inport  Port=7
  U : Inport  Port=8
  Xtrim : Inport  Port=9
  L : Inport  Port=10
  M : Inport  Port=11
  P : Inport  Port=12
  "\tCX" : Product  Multiplication=Matrix(*)
  AX : Product  Multiplication=Matrix(*)
  BU : Product  Multiplication=Matrix(*)
  Convert 1-D to 2-D : dspsigattribs/Convert 1-D to 2-D  M=10  N=1  frameBasedOut=off
      settings: SourceProductName=DSP System Toolbox  SourceProductBaseCode=DS
  Convert 1-D to 2-D1 : dspsigattribs/Convert 1-D to 2-D  M=2  N=1  frameBasedOut=off
      settings: SourceProductName=DSP System Toolbox  SourceProductBaseCode=DS
  DU : Product  Multiplication=Matrix(*)
  Delay : Delay  DelayLength=1  InitialConditionSource=Input port
      settings: InputPortMap=u0,p4
  KY : Product  Multiplication=Matrix(*)
  LP : Product  Multiplication=Matrix(*)
  MATLAB Function : MATLAB Function  TreatAsAtomicUnit=on
  MP : Product  Multiplication=Matrix(*)
  Minus : Sum  Inputs=+-
  Minus1 : Sum
  Minus2 : Sum  Inputs=+-
  Minus3 : Sum  Inputs=++++
  Minus4 : Sum  Inputs=+++
  X_es : Outport
  Y_es : Outport  Port=2
  Y_error : Outport  Port=3
  wires:
  MATLAB Function/1(y) -> KY/2, Y_error/1
  Minus2/1 -> MATLAB Function/1(u)
  Convert 1-D to 2-D1/1 -> Delay/2
  x0/1 -> Convert 1-D to 2-D1/1
  Convert 1-D to 2-D/1 -> MP/2, LP/2
  P/1 -> Convert 1-D to 2-D/1
  MP/1 -> Minus4/3
  LP/1 -> Minus3/4
  M/1 -> MP/1
  L/1 -> LP/1
  Minus4/1 -> Minus2/2, Y_es/1
  KY/1 -> Minus3/1
  U/1 -> BU/2, DU/2
  Y/1 -> Minus2/1
  DU/1 -> Minus4/2
  "\tCX"/1 -> Minus4/1
  BU/1 -> Minus3/3
  A/1 -> AX/1
  B/1 -> BU/1
  C/1 -> "\tCX"/1
  D/1 -> DU/1
  K/1 -> KY/1
  Xtrim/1 -> Minus1/2, Minus/2
  Delay/1 -> Minus/1, X_es/1
  Minus/1 -> AX/2, "\tCX"/2
  AX/1 -> Minus3/2
  Minus3/1 -> Minus1/1
  Minus1/1 -> Delay/1

== system kalman_estimate_MM/PIECE kalman1/kalman filter1 ==
  A : Inport
  B : Inport  Port=2
  C : Inport  Port=3
  D : Inport  Port=4
  K : Inport  Port=5
  x0 : Inport  Port=6
  Y : Inport  Port=7
  U : Inport  Port=8
  Xtrim : Inport  Port=9
  L : Inport  Port=10
  M : Inport  Port=11
  P : Inport  Port=12
  "\tCX" : Product  Multiplication=Matrix(*)
  AX : Product  Multiplication=Matrix(*)
  BU : Product  Multiplication=Matrix(*)
  Convert 1-D to 2-D : dspsigattribs/Convert 1-D to 2-D  M=10  N=1  frameBasedOut=off
      settings: SourceProductName=DSP System Toolbox  SourceProductBaseCode=DS
  Convert 1-D to 2-D1 : dspsigattribs/Convert 1-D to 2-D  M=2  N=1  frameBasedOut=off
      settings: SourceProductName=DSP System Toolbox  SourceProductBaseCode=DS
  DU : Product  Multiplication=Matrix(*)
  Delay : Delay  DelayLength=1  InitialConditionSource=Input port
      settings: InputPortMap=u0,p4
  KY : Product  Multiplication=Matrix(*)
  LP : Product  Multiplication=Matrix(*)
  MATLAB Function : MATLAB Function  TreatAsAtomicUnit=on
  MP : Product  Multiplication=Matrix(*)
  Minus : Sum  Inputs=+-
  Minus1 : Sum
  Minus2 : Sum  Inputs=+-
  Minus3 : Sum  Inputs=++++
  Minus4 : Sum  Inputs=+++
  X_es : Outport
  Y_es : Outport  Port=2
  Y_error : Outport  Port=3
  wires:
  MATLAB Function/1(y) -> KY/2, Y_error/1
  Minus2/1 -> MATLAB Function/1(u)
  Convert 1-D to 2-D1/1 -> Delay/2
  x0/1 -> Convert 1-D to 2-D1/1
  Convert 1-D to 2-D/1 -> MP/2, LP/2
  P/1 -> Convert 1-D to 2-D/1
  MP/1 -> Minus4/3
  LP/1 -> Minus3/4
  M/1 -> MP/1
  L/1 -> LP/1
  Minus4/1 -> Minus2/2, Y_es/1
  KY/1 -> Minus3/1
  U/1 -> BU/2, DU/2
  Y/1 -> Minus2/1
  DU/1 -> Minus4/2
  "\tCX"/1 -> Minus4/1
  BU/1 -> Minus3/3
  A/1 -> AX/1
  B/1 -> BU/1
  C/1 -> "\tCX"/1
  D/1 -> DU/1
  K/1 -> KY/1
  Xtrim/1 -> Minus1/2, Minus/2
  Delay/1 -> Minus/1, X_es/1
  Minus/1 -> AX/2, "\tCX"/2
  AX/1 -> Minus3/2
  Minus3/1 -> Minus1/1
  Minus1/1 -> Delay/1

== system kalman_estimate_MM/PWL/kalman filter1 ==
  A : Inport
  B : Inport  Port=2
  C : Inport  Port=3
  D : Inport  Port=4
  K : Inport  Port=5
  x0 : Inport  Port=6
  U : Inport  Port=7
  Xtrim : Inport  Port=8
  L : Inport  Port=9
  M : Inport  Port=10
  P : Inport  Port=11
  "\tCX" : Product  Multiplication=Matrix(*)
  AX : Product  Multiplication=Matrix(*)
  BU : Product  Multiplication=Matrix(*)
  Convert 1-D to 2-D : dspsigattribs/Convert 1-D to 2-D  M=10  N=1  frameBasedOut=off
      settings: SourceProductName=DSP System Toolbox  SourceProductBaseCode=DS
  Convert 1-D to 2-D1 : dspsigattribs/Convert 1-D to 2-D  M=2  N=1  frameBasedOut=off
      settings: SourceProductName=DSP System Toolbox  SourceProductBaseCode=DS
  DU : Product  Multiplication=Matrix(*)
  Delay : Delay  DelayLength=1  InitialConditionSource=Input port
      settings: InputPortMap=u0,p4
  LP : Product  Multiplication=Matrix(*)
  MP : Product  Multiplication=Matrix(*)
  Minus : Sum  Inputs=+-
  Minus1 : Sum
  Minus3 : Sum  Inputs=+++
  Minus4 : Sum  Inputs=+++
  X_es : Outport
  Y_es : Outport  Port=2
  wires:
  Minus1/1 -> Delay/1
  Minus3/1 -> Minus1/1
  AX/1 -> Minus3/2
  Minus/1 -> "\tCX"/2, AX/2
  Delay/1 -> X_es/1, Minus/1
  Xtrim/1 -> Minus/2, Minus1/2
  D/1 -> DU/1
  C/1 -> "\tCX"/1
  B/1 -> BU/1
  A/1 -> AX/1
  "\tCX"/1 -> Minus4/1
  DU/1 -> Minus4/2
  U/1 -> DU/2, BU/2
  Minus4/1 -> Y_es/1
  L/1 -> LP/1
  M/1 -> MP/1
  MP/1 -> Minus4/3
  P/1 -> Convert 1-D to 2-D/1
  Convert 1-D to 2-D/1 -> LP/2, MP/2
  x0/1 -> Convert 1-D to 2-D1/1
  Convert 1-D to 2-D1/1 -> Delay/2
  BU/1 -> Minus3/1
  LP/1 -> Minus3/3

== system kalman_estimate_MM/act_PIECE kalman/kalman filter1 ==
  A : Inport
  B : Inport  Port=2
  C : Inport  Port=3
  D : Inport  Port=4
  K : Inport  Port=5
  x0 : Inport  Port=6
  Y : Inport  Port=7
  U : Inport  Port=8
  Xtrim : Inport  Port=9
  "\tCX" : Product  Multiplication=Matrix(*)
  AX : Product  Multiplication=Matrix(*)
  BU : Product  Multiplication=Matrix(*)
  Convert 1-D to 2-D1 : dspsigattribs/Convert 1-D to 2-D  M=2  N=1  frameBasedOut=off
      settings: SourceProductName=DSP System Toolbox  SourceProductBaseCode=DS
  DU : Product  Multiplication=Matrix(*)
  Delay : Delay  DelayLength=1  InitialConditionSource=Input port
      settings: InputPortMap=u0,p4
  KY : Product  Multiplication=Matrix(*)
  MATLAB Function : MATLAB Function  TreatAsAtomicUnit=on
  Minus : Sum  Inputs=+-
  Minus1 : Sum
  Minus2 : Sum  Inputs=+-
  Minus3 : Sum  Inputs=+++
  Minus4 : Sum
  X_es : Outport
  Y_es : Outport  Port=2
  Y_error : Outport  Port=3
  wires:
  MATLAB Function/1(y) -> KY/2, Y_error/1
  Minus2/1 -> MATLAB Function/1(u)
  Convert 1-D to 2-D1/1 -> Delay/2
  x0/1 -> Convert 1-D to 2-D1/1
  Minus4/1 -> Minus2/2, Y_es/1
  KY/1 -> Minus3/1
  U/1 -> BU/2, DU/2
  Y/1 -> Minus2/1
  DU/1 -> Minus4/2
  "\tCX"/1 -> Minus4/1
  BU/1 -> Minus3/3
  A/1 -> AX/1
  B/1 -> BU/1
  C/1 -> "\tCX"/1
  D/1 -> DU/1
  K/1 -> KY/1
  Xtrim/1 -> Minus1/2, Minus/2
  Delay/1 -> Minus/1, X_es/1
  Minus/1 -> AX/2, "\tCX"/2
  AX/1 -> Minus3/2
  Minus3/1 -> Minus1/1
  Minus1/1 -> Delay/1

== system kalman_estimate_MM/act_PWL/kalman filter1 ==
  A : Inport
  B : Inport  Port=2
  C : Inport  Port=3
  D : Inport  Port=4
  x0 : Inport  Port=5
  U : Inport  Port=6
  Xtrim : Inport  Port=7
  "\tCX" : Product  Multiplication=Matrix(*)
  AX : Product  Multiplication=Matrix(*)
  BU : Product  Multiplication=Matrix(*)
  Convert 1-D to 2-D1 : dspsigattribs/Convert 1-D to 2-D  M=2  N=1  frameBasedOut=off
      settings: SourceProductName=DSP System Toolbox  SourceProductBaseCode=DS
  DU : Product  Multiplication=Matrix(*)
  Delay : Delay  DelayLength=1  InitialConditionSource=Input port
      settings: InputPortMap=u0,p4
  Minus : Sum  Inputs=+-
  Minus1 : Sum
  Minus3 : Sum
  Minus4 : Sum
  X_es : Outport
  Y_es : Outport  Port=2
  wires:
  BU/1 -> Minus3/1
  Convert 1-D to 2-D1/1 -> Delay/2
  x0/1 -> Convert 1-D to 2-D1/1
  Minus4/1 -> Y_es/1
  U/1 -> BU/2, DU/2
  DU/1 -> Minus4/2
  "\tCX"/1 -> Minus4/1
  A/1 -> AX/1
  B/1 -> BU/1
  C/1 -> "\tCX"/1
  D/1 -> DU/1
  Xtrim/1 -> Minus1/2, Minus/2
  Delay/1 -> Minus/1, X_es/1
  Minus/1 -> AX/2, "\tCX"/2
  AX/1 -> Minus3/2
  Minus3/1 -> Minus1/1
  Minus1/1 -> Delay/1

== system kalman_estimate_MM/act_PWL_model/kalman filter1 ==
  A : Inport
  B : Inport  Port=2
  C : Inport  Port=3
  D : Inport  Port=4
  x0 : Inport  Port=5
  U : Inport  Port=6
  Xtrim : Inport  Port=7
  "\tCX" : Product  Multiplication=Matrix(*)
  AX : Product  Multiplication=Matrix(*)
  BU : Product  Multiplication=Matrix(*)
  Convert 1-D to 2-D1 : dspsigattribs/Convert 1-D to 2-D  M=2  N=1  frameBasedOut=off
      settings: SourceProductName=DSP System Toolbox  SourceProductBaseCode=DS
  DU : Product  Multiplication=Matrix(*)
  Delay : Delay  DelayLength=1  InitialConditionSource=Input port
      settings: InputPortMap=u0,p4
  Minus : Sum  Inputs=+-
  Minus1 : Sum
  Minus3 : Sum
  Minus4 : Sum
  X_es : Outport
  Y_es : Outport  Port=2
  wires:
  Minus1/1 -> Delay/1
  Minus3/1 -> Minus1/1
  AX/1 -> Minus3/2
  Minus/1 -> "\tCX"/2, AX/2
  Delay/1 -> X_es/1, Minus/1
  Xtrim/1 -> Minus/2, Minus1/2
  D/1 -> DU/1
  C/1 -> "\tCX"/1
  B/1 -> BU/1
  A/1 -> AX/1
  "\tCX"/1 -> Minus4/1
  DU/1 -> Minus4/2
  U/1 -> DU/2, BU/2
  Minus4/1 -> Y_es/1
  x0/1 -> Convert 1-D to 2-D1/1
  Convert 1-D to 2-D1/1 -> Delay/2
  BU/1 -> Minus3/1

== system kalman_estimate_MM/com_PIECE kalman/kalman filter1 ==
  A : Inport
  B : Inport  Port=2
  C : Inport  Port=3
  D : Inport  Port=4
  K : Inport  Port=5
  x0 : Inport  Port=6
  Y : Inport  Port=7
  U : Inport  Port=8
  Xtrim : Inport  Port=9
  "\tCX" : Product  Multiplication=Matrix(*)
  AX : Product  Multiplication=Matrix(*)
  BU : Product  Multiplication=Matrix(*)
  Convert 1-D to 2-D1 : dspsigattribs/Convert 1-D to 2-D  M=2  N=1  frameBasedOut=off
      settings: SourceProductName=DSP System Toolbox  SourceProductBaseCode=DS
  DU : Product  Multiplication=Matrix(*)
  Delay : Delay  DelayLength=1  InitialConditionSource=Input port
      settings: InputPortMap=u0,p4
  KY : Product  Multiplication=Matrix(*)
  MATLAB Function : MATLAB Function  TreatAsAtomicUnit=on
  Minus : Sum  Inputs=+-
  Minus1 : Sum
  Minus2 : Sum  Inputs=+-
  Minus3 : Sum  Inputs=+++
  Minus4 : Sum
  X_es : Outport
  Y_es : Outport  Port=2
  Y_error : Outport  Port=3
  wires:
  MATLAB Function/1(y) -> KY/2, Y_error/1
  Minus2/1 -> MATLAB Function/1(u)
  Convert 1-D to 2-D1/1 -> Delay/2
  x0/1 -> Convert 1-D to 2-D1/1
  Minus4/1 -> Minus2/2, Y_es/1
  KY/1 -> Minus3/1
  U/1 -> BU/2, DU/2
  Y/1 -> Minus2/1
  DU/1 -> Minus4/2
  "\tCX"/1 -> Minus4/1
  BU/1 -> Minus3/3
  A/1 -> AX/1
  B/1 -> BU/1
  C/1 -> "\tCX"/1
  D/1 -> DU/1
  K/1 -> KY/1
  Xtrim/1 -> Minus1/2, Minus/2
  Delay/1 -> Minus/1, X_es/1
  Minus/1 -> AX/2, "\tCX"/2
  AX/1 -> Minus3/2
  Minus3/1 -> Minus1/1
  Minus1/1 -> Delay/1

== system kalman_estimate_MM/component_PWL/kalman filter1 ==
  A : Inport
  B : Inport  Port=2
  C : Inport  Port=3
  D : Inport  Port=4
  x0 : Inport  Port=5
  U : Inport  Port=6
  Xtrim : Inport  Port=7
  "\tCX" : Product  Multiplication=Matrix(*)
  AX : Product  Multiplication=Matrix(*)
  BU : Product  Multiplication=Matrix(*)
  Convert 1-D to 2-D1 : dspsigattribs/Convert 1-D to 2-D  M=2  N=1  frameBasedOut=off
      settings: SourceProductName=DSP System Toolbox  SourceProductBaseCode=DS
  DU : Product  Multiplication=Matrix(*)
  Delay : Delay  DelayLength=1  InitialConditionSource=Input port
      settings: InputPortMap=u0,p4
  Minus : Sum  Inputs=+-
  Minus1 : Sum
  Minus3 : Sum
  Minus4 : Sum
  X_es : Outport
  Y_es : Outport  Port=2
  wires:
  BU/1 -> Minus3/1
  Convert 1-D to 2-D1/1 -> Delay/2
  x0/1 -> Convert 1-D to 2-D1/1
  Minus4/1 -> Y_es/1
  U/1 -> BU/2, DU/2
  DU/1 -> Minus4/2
  "\tCX"/1 -> Minus4/1
  A/1 -> AX/1
  B/1 -> BU/1
  C/1 -> "\tCX"/1
  D/1 -> DU/1
  Xtrim/1 -> Minus1/2, Minus/2
  Delay/1 -> Minus/1, X_es/1
  Minus/1 -> AX/2, "\tCX"/2
  AX/1 -> Minus3/2
  Minus3/1 -> Minus1/1
  Minus1/1 -> Delay/1

== system kalman_estimate_MM/component_PWL1/kalman filter1 ==
  A : Inport
  B : Inport  Port=2
  C : Inport  Port=3
  D : Inport  Port=4
  x0 : Inport  Port=5
  U : Inport  Port=6
  Xtrim : Inport  Port=7
  "\tCX" : Product  Multiplication=Matrix(*)
  AX : Product  Multiplication=Matrix(*)
  BU : Product  Multiplication=Matrix(*)
  Convert 1-D to 2-D1 : dspsigattribs/Convert 1-D to 2-D  M=2  N=1  frameBasedOut=off
      settings: SourceProductName=DSP System Toolbox  SourceProductBaseCode=DS
  DU : Product  Multiplication=Matrix(*)
  Delay : Delay  DelayLength=1  InitialConditionSource=Input port
      settings: InputPortMap=u0,p4
  Minus : Sum  Inputs=+-
  Minus1 : Sum
  Minus3 : Sum
  Minus4 : Sum
  X_es : Outport
  Y_es : Outport  Port=2
  wires:
  BU/1 -> Minus3/1
  Convert 1-D to 2-D1/1 -> Delay/2
  x0/1 -> Convert 1-D to 2-D1/1
  Minus4/1 -> Y_es/1
  U/1 -> BU/2, DU/2
  DU/1 -> Minus4/2
  "\tCX"/1 -> Minus4/1
  A/1 -> AX/1
  B/1 -> BU/1
  C/1 -> "\tCX"/1
  D/1 -> DU/1
  Xtrim/1 -> Minus1/2, Minus/2
  Delay/1 -> Minus/1, X_es/1
  Minus/1 -> AX/2, "\tCX"/2
  AX/1 -> Minus3/2
  Minus3/1 -> Minus1/1
  Minus1/1 -> Delay/1

== system kalman_estimate_MM/health_PWL/kalman filter1 ==
  A : Inport
  B : Inport  Port=2
  C : Inport  Port=3
  D : Inport  Port=4
  K : Inport  Port=5
  x0 : Inport  Port=6
  U : Inport  Port=7
  Xtrim : Inport  Port=8
  L : Inport  Port=9
  M : Inport  Port=10
  P : Inport  Port=11
  "\tCX" : Product  Multiplication=Matrix(*)
  AX : Product  Multiplication=Matrix(*)
  BU : Product  Multiplication=Matrix(*)
  Convert 1-D to 2-D : dspsigattribs/Convert 1-D to 2-D  M=10  N=1  frameBasedOut=off
      settings: SourceProductName=DSP System Toolbox  SourceProductBaseCode=DS
  Convert 1-D to 2-D1 : dspsigattribs/Convert 1-D to 2-D  M=2  N=1  frameBasedOut=off
      settings: SourceProductName=DSP System Toolbox  SourceProductBaseCode=DS
  DU : Product  Multiplication=Matrix(*)
  Delay : Delay  DelayLength=1  InitialConditionSource=Input port
      settings: InputPortMap=u0,p4
  LP : Product  Multiplication=Matrix(*)
  MP : Product  Multiplication=Matrix(*)
  Minus : Sum  Inputs=+-
  Minus1 : Sum
  Minus3 : Sum  Inputs=+++
  Minus4 : Sum  Inputs=+++
  X_es : Outport
  Y_es : Outport  Port=2
  wires:
  Minus1/1 -> Delay/1
  Minus3/1 -> Minus1/1
  AX/1 -> Minus3/2
  Minus/1 -> "\tCX"/2, AX/2
  Delay/1 -> X_es/1, Minus/1
  Xtrim/1 -> Minus/2, Minus1/2
  D/1 -> DU/1
  C/1 -> "\tCX"/1
  B/1 -> BU/1
  A/1 -> AX/1
  "\tCX"/1 -> Minus4/1
  DU/1 -> Minus4/2
  U/1 -> DU/2, BU/2
  Minus4/1 -> Y_es/1
  L/1 -> LP/1
  M/1 -> MP/1
  MP/1 -> Minus4/3
  P/1 -> Convert 1-D to 2-D/1
  Convert 1-D to 2-D/1 -> LP/2, MP/2
  x0/1 -> Convert 1-D to 2-D1/1
  Convert 1-D to 2-D1/1 -> Delay/2
  BU/1 -> Minus3/1
  LP/1 -> Minus3/3
